simulink model "pll_model_on_blocks"  (R2012b)
settings: Solver=FixedStepDiscrete  StartTime=0.0  StopTime=0.2  RelTol=1e-3
InitFcn:
  | clear_simulation
StartFcn:
  | open_scopes
settings Model: Creator=Tomasz  LastModifiedBy=Tomasz
settings SFSimCC: SimBuildMode=sf_make_clean

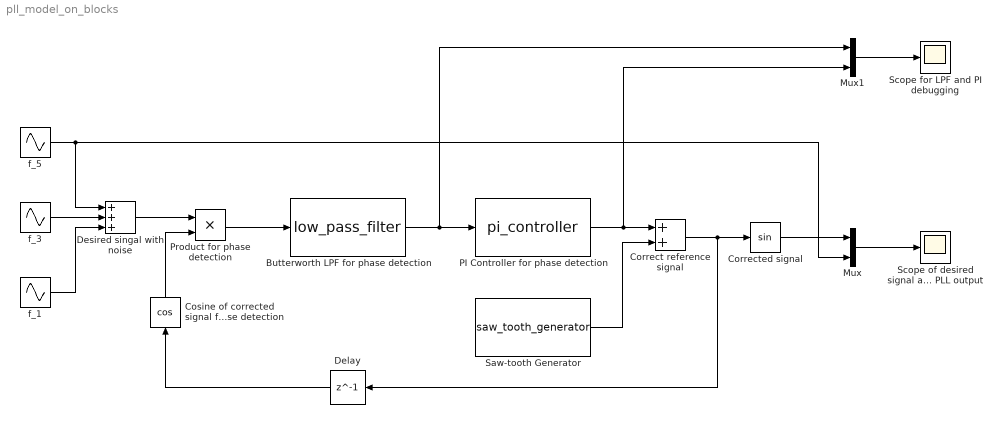
== system pll_model_on_blocks ==
  Butterworth LPF for phase detection : S-Function  InitFcn=try, set_param(gcb,'FunctionName','low_pass_filter'), end  FunctionName=low_pass_filter  SFunctionModules=low_pass_filter_wrapper butterworth  EnableBusSupport=off  mask(S-Function Builder){}
      mask help: Simulink:masks:SFunctionBuilder_MD
      mask init:
      | val = [[.9  0.75 0.75 1 1 .9 .9 1]',[1 1 0.75 0.75 .9 .9 1 .9]'];try , sys = get_param(gcb,'SfunBuilderFcnName');if isempty(sys), sys = get_param(gcb,'FunctionName'); end,catch, sys = get_param(gcb,'FunctionName'); end
      settings: CopyFcn=set_param(gcbh,'LinkStatus','none')  PreSaveFcn=try, set_param(gcb,'FunctionName','low_pass_filter'), end  OpenFcn=sfunctionwizard(gcbh)
      mask Display: plot(val(:,1),val(:,2)),disp(sys), port_label('input',1,'u'), port_label('output',1,'y')
  Correct reference signal : Sum
  Corrected signal : Trigonometry
  Cosine of corrected signal for phase detection : Trigonometry  Operator=cos
  Delay : Delay  DelayLength=1
  Desired singal with noise : Sum  Inputs=+++
  Mux : Mux  Inputs=2
  Mux1 : Mux  Inputs=2
  PI Controller for phase detection : S-Function  InitFcn=try, set_param(gcb,'FunctionName','pi_controller'), end  FunctionName=pi_controller  Parameters=0.008,0.3  SFunctionModules=pi_controller_wrapper  EnableBusSupport=off  mask(S-Function Builder){}
      mask help: Simulink:masks:SFunctionBuilder_MD
      mask init: same as pll_model_on_blocks/Butterworth LPF for phase detection
      settings: CopyFcn=set_param(gcbh,'LinkStatus','none')  PreSaveFcn=try, set_param(gcb,'FunctionName','pi_controller'), end  OpenFcn=sfunctionwizard(gcbh)
      mask Display: plot(val(:,1),val(:,2)),disp(sys), port_label('input',1,'u'), port_label('output',1,'y')
  Product for phase detection : Product  RndMeth=Zero
  Saw-tooth Generator : S-Function  InitFcn=try, set_param(gcb,'FunctionName','saw_tooth_generator'), end  FunctionName=saw_tooth_generator  SFunctionModules=saw_tooth_generator_wrapper  EnableBusSupport=off  mask(S-Function Builder){}
      mask help: Simulink:masks:SFunctionBuilder_MD
      mask init: same as pll_model_on_blocks/Butterworth LPF for phase detection
      settings: CopyFcn=set_param(gcbh,'LinkStatus','none')  PreSaveFcn=try, set_param(gcb,'FunctionName','saw_tooth_generator'), end  OpenFcn=sfunctionwizard(gcbh)
      mask Display: plot(val(:,1),val(:,2)),disp(sys), port_label('output',1,'y')
  "Scope for LPF and PI debugging " : Scope
      settings: ShowLegends=on  YMin=-0.1  YMax=1  MaxDataPoints=1e4
  Scope of desired signal and PLL output : Scope
      settings: TickLabels=on  ShowLegends=on  YMin=-1  YMax=1  MaxDataPoints=1e4
  f_1 : Sin  Frequency=50 * 2 * pi  Phase=5 / 180 * pi  SampleTime=1e-4
  f_3 : Sin  Frequency=150 * 2 * pi  Phase=10 / 180 * pi  SampleTime=1e-4
  f_5 : Sin  Frequency=250 * 2 * pi  Phase=30 / 180 * pi  SampleTime=1e-4
  wires:
  f_5/1 -> Desired singal with noise/1, Mux/2
  f_3/1 -> Desired singal with noise/2
  f_1/1 -> Desired singal with noise/3
  Desired singal with noise/1 -> Product for phase detection/1
  Product for phase detection/1 -> Butterworth LPF for phase detection/1
  Butterworth LPF for phase detection/1 -> Mux1/1, PI Controller for phase detection/1
  PI Controller for phase detection/1 -> Mux1/2, Correct reference signal/1
  Saw-tooth Generator/1 -> Correct reference signal/2
  Mux/1 -> Scope of desired signal and PLL output/1
  Correct reference signal/1 -> Delay/1, Corrected signal/1
  Corrected signal/1 -> Mux/1
  Cosine of corrected signal for phase detection/1 -> Product for phase detection/2
  Delay/1 -> Cosine of corrected signal for phase detection/1
  Mux1/1 -> "Scope for LPF and PI debugging "/1
